simulink library "ddm"  (R2021b)
settings: Solver=VariableStepAuto  StartTime=0.0  StopTime=10.0  RelTol=1e-3
undefined symbols (not defined in the file): ADDM_FrTMTqDev_X_Nm, ADDM_RrTMTqDev_X_Nm, ENUM_ADASACCSTA_ERROR, ENUM_ADASACCSTA_OFF, ENUM_ADASACCSTA_STANDBY, ENUM_ALLOWMOV_ALLOWREADY, ENUM_APS, ENUM_BRKSTA_ERROR, ENUM_BRKSTA_OFF, ENUM_BRKSTA_ON, ENUM_BRKSW_INVALID, ENUM_BRKSW_OFF, ENUM_BRKSW_ON, ENUM_CHGPREACTERRSTA_OBCPRE, ENUM_DCDCFAULTSTA_ANYFAULTLV1, ENUM_DCDCFAULTSTA_ANYFAULTLV2, ENUM_DRIVETRAIN_AWD, ENUM_DRIVETRAIN_FWD, ENUM_DRIVETRAIN_RWD, ENUM_EDUDRTSTA_NORMAL, ENUM_EPBERROR_FAILED, ENUM_EPBSTA_APPLIED, ENUM_EPBSTA_RELEASED, ENUM_ESCAPSSta_APSUNAVAILABLE, ENUM_GEARACTUALPOSN_INVALID, ENUM_GEARACTUALPOSN_P, ENUM_HVBATTREADYPRE_READY, ENUM_HWRESETSTA_HWRESETING, ENUM_MCUWARN_LV0, ENUM_MCUWARN_LV1, ENUM_MCUWARN_LV2, ENUM_MCUWARN_LV3, ENUM_MCUWARN_NOERROR, ENUM_OBCFAULTSTA_ANYFAULT, ENUM_PAS_R2F2, ENUM_PDFAULT_BATTPDFAIL, ENUM_PDFAULT_DCDCDISABLE, ENUM_PDFAULT_MCUDISABLE, ENUM_PDFAULT_MCUDISCHRG, ENUM_POWERSTA_OFF, ENUM_POWERSTA_ON, ENUM_POWERSTA_READY, ENUM_POWERSTA_STANDBY, ENUM_PRESSINDI_LOW, ENUM_PUFAULT_BATTUPFAIL, ENUM_PUFAULT_DCDCENABLEFAIL, ENUM_PUFAULT_PRECHRGCHKFAIL, ENUM_PUFAULT_SAFETYCHKFAIL, ENUM_PWRSTASW_OFF, ENUM_PWRSTASW_OFFA, ENUM_PWRSTASW_OFFCHVCHRG, ENUM_PWRSTASW_OFFCLVCHRG, ENUM_PWRSTASW_ON, ENUM_PWRSTASW_ONHVCHRG, ENUM_PWRSTASW_READY, ENUM_PWRSTASW_STANDBY, ENUM_RAPSErrWarnSta_NORMAL, ENUM_RAPSErrWarnSta_RAPSERRLV1, ENUM_SHIFTCOMMAND_P, ENUM_SHIFTERERRSTA_PBUTTONFAILURE ... (+471)
libraries: hcu_lib x540, simulink x3
(part 22 of 26)

== system ddm/DDM/DDM/PMM/power up and power down/BMS ready fail ==
  note: Test Pass Criteria
  note: Release Condition After Decision
  note: Diagnostics and Fault Handling
  note: Test Detection Criteria
  task_time_s : Inport
  VPMM_PowerSta_enum : Inport  Port=2
  VPMM_PwrStaSW_enum : Inport  Port=3
  VINP_BMSREADY_flg : Inport  Port=4
  VPMM_PowerUpFault_enum : Inport  Port=5
  DTC_clear_request : Inport  Port=6
  Constant : Constant  Value=ENUM_PUFAULT_BATTUPFAIL
  Constant1 : Constant  Value=ENUM_PWRSTASW_OFF
  Constant12 : Constant  Value=ENUM_PWRSTASW_OFF
  Constant13 : Constant  Value=FALSE
  Constant14 : Constant  Value=ZERO_INT
  Constant17 : Constant  Value=KDDM_PwrUpDnDiagnosisOffSW_flg
  Constant18 : Constant  Value=KDDM_BMSRdyPassTO_s
  Constant22 : Constant  Value=ENUM_POWERSTA_OFF
  Constant26 : Constant  Value=KDDM_BMSRdyDTC_cnt
  Constant28 : Constant  Value=KDDM_BMSRdyDTC_cnt
  Constant29 : Constant  Value=FALSE
  Constant41 : Constant  Value=KDDM_BMSRdyDetTO_s
  Constant6 : Constant  Value=TRUE
  Constant7 : Constant  Value=ENUM_POWERSTA_STANDBY
  Constant9 : Constant  Value=KDDM_BMSRdyPassTO_s
  DTC_Couter1 : hcu_lib/Basic_Blocks/DTC_Couter
  DTC_Info : hcu_lib/Basic_Blocks/DTC_Info
  Equal1 : RelationalOperator  Operator===  OutDataTypeStr=boolean  RndMeth=Simplest
  Equal2 : RelationalOperator  Operator=~=  OutDataTypeStr=boolean  RndMeth=Simplest
  Equal4 : RelationalOperator  Operator=~=  OutDataTypeStr=boolean  RndMeth=Simplest
  Equal7 : RelationalOperator  OutDataTypeStr=boolean  RndMeth=Simplest
  Equal8 : RelationalOperator  Operator===  OutDataTypeStr=boolean  RndMeth=Simplest
  Equal9 : RelationalOperator  Operator===  OutDataTypeStr=boolean  RndMeth=Simplest
  Logical Operator13 : Logic  Operator=NOT  AllPortsSameDT=off  OutDataTypeStr=boolean
  Logical Operator14 : Logic  Operator=OR  Inputs=4  AllPortsSameDT=off  OutDataTypeStr=boolean
  Logical Operator16 : Logic  AllPortsSameDT=off  OutDataTypeStr=boolean
  Logical Operator4 : Logic  Operator=NOT  AllPortsSameDT=off  OutDataTypeStr=boolean
  Logical Operator5 : Logic  AllPortsSameDT=off  OutDataTypeStr=boolean
  Relational Operator1 : RelationalOperator  Operator=>  OutDataTypeStr=boolean  RndMeth=Simplest
  Switch1 : Switch  Criteria=u2 ~= 0
  Switch3 : Switch  Criteria=u2 ~= 0
  Switch6 : Switch  Criteria=u2 ~= 0
  Terminator : Terminator
  Test Detection Criteria1 : hcu_lib/Basic_Blocks/Test Detection Criteria
  Timer2 : hcu_lib/Basic_Blocks/Timer
  Unit Delay1 : UnitDelay  SampleTime=-1  HasFrameUpgradeWarning=on
  VDDM_BMSRdyDTC_raw32 : Outport
  VDDM_BMSRdyCFS_flg : Outport  Port=2
  wires:
  [VDDM_BMSRdyCFS_flg] -> VDDM_BMSRdyCFS_flg/1
  Constant12/1 -> Equal4/2
  Constant9/1 -> Timer2/4
  [VPMM_PwrStaSW_enum] -> Equal4/1
  Timer2/1 -> Equal7/1
  Switch1/1 -> Logical Operator13/1, Timer2/2
  Constant6/1 -> Switch1/3
  Constant22/1 -> Equal8/2
  Logical Operator16/1 -> Logical Operator14/1
  Equal8/1 -> Logical Operator16/1
  Constant14/1 -> Relational Operator1/2
  Constant28/1 -> Test Detection Criteria1/3
  Constant18/1 -> Equal7/2
  [task_time_s] -> Timer2/3
  Constant41/1 -> Test Detection Criteria1/4
  [VDDM_BMSRdyCFSRls_flg] -> DTC_Couter1/2
  Constant26/1 -> DTC_Couter1/3
  Logical Operator13/1 -> Timer2/1
  Relational Operator1/1 -> Terminator/1  "VDDM_BMSRdyDFS_flg"
  DTC_Couter1/2 -> Relational Operator1/1  "VDDM_BMSRdyDTC_cnt"
  [VDDM_BMSRdyDet_flg] -> DTC_Couter1/1
  Equal9/1 -> Logical Operator16/2
  Switch6/1 -> Test Detection Criteria1/1
  Constant17/1 -> Logical Operator14/4
  [task_time_s] -> Test Detection Criteria1/2
  Unit Delay1/1 -> Equal8/1
  Constant7/1 -> Equal9/2
  Constant29/1 -> Switch6/1
  Constant13/1 -> Switch3/3
  Logical Operator14/1 -> [VDDM_BMSRdyCFSRls_flg]  "VDDM_BMSRdyCFSRls_flg"
  [VDDM_BMSRdyPass_flg] -> Logical Operator14/3
  Test Detection Criteria1/1 -> [VDDM_BMSRdyDet_flg]  "VDDM_BMSRdyDet_flg"
  Equal4/1 -> Switch3/2
  [VPMM_PowerSta_enum] -> Equal9/1
  Switch3/1 -> Switch6/3
  [VDDM_BMSRdyCFSRls_flg] -> Switch6/2
  [VPMM_PowerSta_enum] -> Unit Delay1/1
  DTC_Couter1/1 -> [VDDM_BMSRdyCFS_flg]  "VDDM_BMSRdyCFS_flg"
  [VDDM_BMSRdyChk_flg] -> Switch3/1
  Equal7/1 -> [VDDM_BMSRdyPass_flg]  "VDDM_BMSRdyPass_flg"
  [DTC_clear_request] -> Logical Operator14/2
  Equal2/1 -> Switch1/2
  Logical Operator5/1 -> [VDDM_BMSRdyChk_flg]
  VPMM_PowerUpFault_enum/1 -> Equal1/1
  VINP_BMSREADY_flg/1 -> Logical Operator4/1
  Logical Operator4/1 -> Logical Operator5/1
  Equal1/1 -> Logical Operator5/2
  Constant/1 -> Equal1/2
  DTC_clear_request/1 -> [DTC_clear_request]
  VPMM_PowerSta_enum/1 -> [VPMM_PowerSta_enum]
  VPMM_PwrStaSW_enum/1 -> [VPMM_PwrStaSW_enum]
  task_time_s/1 -> [task_time_s]
  DTC_Info/1 -> VDDM_BMSRdyDTC_raw32/1  "VDDM_BMSRdyDTC_raw32"
  [VDDM_BMSRdyCFS_flg] -> DTC_Info/3
  [VDDM_BMSRdyDet_flg] -> DTC_Info/1
  [VDDM_BMSRdyPass_flg] -> DTC_Info/2
  [DTC_clear_request] -> DTC_Info/4
  Constant1/1 -> Equal2/2
  [VPMM_PwrStaSW_enum] -> Equal2/1
  [VDDM_BMSRdyChk_flg] -> Switch1/1

== system ddm/DDM/DDM/PMM/power up and power down/DCDC disable fail ==
  note: Release Condition After Decision
  note: Test Detection Criteria
  note: Diagnostics and Fault Handling
  note: Test Pass Criteria
  task_time_s : Inport
  VPMM_PowerSta_enum : Inport  Port=2
  VPMM_PwrStaSW_enum : Inport  Port=3
  VPMM_PowerDownFault_enum : Inport  Port=4
  DTC_clear_request : Inport  Port=5
  Constant : Constant  Value=ENUM_PDFAULT_DCDCDISABLE
  Constant1 : Constant  Value=ENUM_PWRSTASW_OFF
  Constant12 : Constant  Value=ENUM_PWRSTASW_OFF
  Constant13 : Constant  Value=FALSE
  Constant14 : Constant  Value=ZERO_INT
  Constant18 : Constant  Value=KDDM_DCDCDisDTC_cnt
  Constant2 : Constant  Value=KDDM_PwrUpDnDiagnosisOffSW_flg
  Constant23 : Constant  Value=TRUE
  Constant26 : Constant  Value=KDDM_DCDCDisDTC_cnt
  Constant29 : Constant  Value=FALSE
  Constant3 : Constant  Value=ENUM_POWERSTA_OFF
  Constant4 : Constant  Value=KDDM_DCDCDisPassTO_s
  Constant41 : Constant  Value=KDDM_DCDCDisDetTO_s
  Constant8 : Constant  Value=ENUM_POWERSTA_STANDBY
  Constant9 : Constant  Value=KDDM_DCDCDisPassTO_s
  DTC_Couter1 : hcu_lib/Basic_Blocks/DTC_Couter
  DTC_Info : hcu_lib/Basic_Blocks/DTC_Info
  Equal1 : RelationalOperator  Operator===  OutDataTypeStr=boolean  RndMeth=Simplest
  Equal10 : RelationalOperator  Operator===  OutDataTypeStr=boolean  RndMeth=Simplest
  Equal2 : RelationalOperator  Operator=~=  OutDataTypeStr=boolean  RndMeth=Simplest
  Equal5 : RelationalOperator  Operator=~=  OutDataTypeStr=boolean  RndMeth=Simplest
  Equal8 : RelationalOperator  OutDataTypeStr=boolean  RndMeth=Simplest
  Equal9 : RelationalOperator  Operator===  OutDataTypeStr=boolean  RndMeth=Simplest
  Logical Operator13 : Logic  Operator=NOT  AllPortsSameDT=off  OutDataTypeStr=boolean
  Logical Operator14 : Logic  Operator=OR  Inputs=4  AllPortsSameDT=off  OutDataTypeStr=boolean
  Logical Operator16 : Logic  AllPortsSameDT=off  OutDataTypeStr=boolean
  Relational Operator1 : RelationalOperator  Operator=>  OutDataTypeStr=boolean  RndMeth=Simplest
  Switch1 : Switch  Criteria=u2 ~= 0
  Switch3 : Switch  Criteria=u2 ~= 0
  Switch6 : Switch  Criteria=u2 ~= 0
  Terminator : Terminator
  Test Detection Criteria1 : hcu_lib/Basic_Blocks/Test Detection Criteria
  Timer2 : hcu_lib/Basic_Blocks/Timer
  Unit Delay1 : UnitDelay  SampleTime=-1  HasFrameUpgradeWarning=on
  VDDM_DCDCDisDTC_raw32 : Outport
  VDDM_DCDCDisCFS_flg : Outport  Port=2
  wires:
  [VDDM_DCDCDisCFS_flg] -> VDDM_DCDCDisCFS_flg/1
  Constant1/1 -> Equal2/2
  Constant23/1 -> Switch1/3
  [VPMM_PwrStaSW_enum] -> Equal2/1
  Equal2/1 -> Switch1/2
  [VDDM_DCDCDisChk_flg] -> Switch1/1
  Constant18/1 -> DTC_Couter1/3
  Timer2/1 -> Equal8/1
  [VPMM_PwrStaSW_enum] -> Equal5/1
  [VDDM_DCDCDisPass_flg] -> Logical Operator14/3
  [VDDM_DCDCDisCFSRls_flg] -> Switch6/2
  Equal9/1 -> Logical Operator16/1
  Constant26/1 -> Test Detection Criteria1/3
  Equal8/1 -> [VDDM_DCDCDisPass_flg]  "VDDM_DCDCDisPass_flg"
  Switch1/1 -> Logical Operator13/1, Timer2/2
  Switch6/1 -> Test Detection Criteria1/1
  Constant41/1 -> Test Detection Criteria1/4
  DTC_Couter1/2 -> Relational Operator1/1  "VDDM_DCDCDisDTC_cnt"
  Equal10/1 -> Logical Operator16/2
  [VDDM_DCDCDisCFSRls_flg] -> DTC_Couter1/2
  Unit Delay1/1 -> Equal9/1
  Constant12/1 -> Equal5/2
  Test Detection Criteria1/1 -> [VDDM_DCDCDisDet_flg]  "VDDM_DCDCDisDet_flg"
  [task_time_s] -> Test Detection Criteria1/2
  [VDDM_DCDCDisDet_flg] -> DTC_Couter1/1
  [task_time_s] -> Timer2/3
  [VPMM_PowerSta_enum] -> Unit Delay1/1
  Constant2/1 -> Logical Operator14/4
  [VPMM_PowerSta_enum] -> Equal10/1
  Constant8/1 -> Equal10/2
  Constant3/1 -> Equal9/2
  Logical Operator13/1 -> Timer2/1
  Logical Operator16/1 -> Logical Operator14/1
  Logical Operator14/1 -> [VDDM_DCDCDisCFSRls_flg]  "VDDM_DCDCDisCFSRls_flg"
  [VDDM_DCDCDisChk_flg] -> Switch3/1
  Relational Operator1/1 -> Terminator/1  "VDDM_DCDCDisDFS_flg"
  Switch3/1 -> Switch6/3
  Constant13/1 -> Switch3/3
  Equal5/1 -> Switch3/2
  Constant29/1 -> Switch6/1
  DTC_Couter1/1 -> [VDDM_DCDCDisCFS_flg]  "VDDM_DCDCDisCFS_flg"
  [DTC_clear_request] -> Logical Operator14/2
  Constant14/1 -> Relational Operator1/2
  Constant4/1 -> Timer2/4
  Constant9/1 -> Equal8/2
  VPMM_PowerSta_enum/1 -> [VPMM_PowerSta_enum]
  VPMM_PwrStaSW_enum/1 -> [VPMM_PwrStaSW_enum]
  task_time_s/1 -> [task_time_s]
  VPMM_PowerDownFault_enum/1 -> Equal1/1
  Constant/1 -> Equal1/2
  DTC_clear_request/1 -> [DTC_clear_request]
  Equal1/1 -> [VDDM_DCDCDisChk_flg]
  DTC_Info/1 -> VDDM_DCDCDisDTC_raw32/1  "VDDM_DCDCDisDTC_raw32"
  [VDDM_DCDCDisPass_flg] -> DTC_Info/2
  [VDDM_DCDCDisCFS_flg] -> DTC_Info/3
  [VDDM_DCDCDisDet_flg] -> DTC_Info/1
  [DTC_clear_request] -> DTC_Info/4

== system ddm/DDM/DDM/PMM/power up and power down/DCDC enable fail ==
  note: Release Condition After Decision
  note: Test Detection Criteria
  note: Test Pass Criteria
  note: Diagnostics and Fault Handling
  task_time_s : Inport
  VPMM_PowerSta_enum : Inport  Port=2
  VPMM_PwrStaSW_enum : Inport  Port=3
  VINP_DCDCEnabled_flg : Inport  Port=4
  VPMM_PowerUpFault_enum : Inport  Port=5
  DTC_clear_request : Inport  Port=6
  Constant : Constant  Value=ENUM_PUFAULT_DCDCENABLEFAIL
  Constant1 : Constant  Value=ENUM_PWRSTASW_OFF
  Constant12 : Constant  Value=ENUM_PWRSTASW_OFF
  Constant13 : Constant  Value=FALSE
  Constant14 : Constant  Value=ZERO_INT
  Constant17 : Constant  Value=KDDM_PwrUpDnDiagnosisOffSW_flg
  Constant18 : Constant  Value=KDDM_DCDCEnaDTC_cnt
  Constant22 : Constant  Value=ENUM_POWERSTA_OFF
  Constant28 : Constant  Value=KDDM_DCDCEnaDTC_cnt
  Constant29 : Constant  Value=FALSE
  Constant3 : Constant  Value=KDDM_DCDCEnaPassTO_s
  Constant41 : Constant  Value=KDDM_DCDCEnaDetTO_s
  Constant6 : Constant  Value=TRUE
  Constant7 : Constant  Value=ENUM_POWERSTA_STANDBY
  Constant9 : Constant  Value=KDDM_DCDCEnaPassTO_s
  DTC_Couter1 : hcu_lib/Basic_Blocks/DTC_Couter
  DTC_Info : hcu_lib/Basic_Blocks/DTC_Info
  Equal1 : RelationalOperator  Operator===  OutDataTypeStr=boolean  RndMeth=Simplest
  Equal2 : RelationalOperator  Operator=~=  OutDataTypeStr=boolean  RndMeth=Simplest
  Equal4 : RelationalOperator  Operator=~=  OutDataTypeStr=boolean  RndMeth=Simplest
  Equal7 : RelationalOperator  OutDataTypeStr=boolean  RndMeth=Simplest
  Equal8 : RelationalOperator  Operator===  OutDataTypeStr=boolean  RndMeth=Simplest
  Equal9 : RelationalOperator  Operator===  OutDataTypeStr=boolean  RndMeth=Simplest
  Logical Operator13 : Logic  Operator=NOT  AllPortsSameDT=off  OutDataTypeStr=boolean
  Logical Operator14 : Logic  Operator=OR  Inputs=4  AllPortsSameDT=off  OutDataTypeStr=boolean
  Logical Operator16 : Logic  AllPortsSameDT=off  OutDataTypeStr=boolean
  Logical Operator4 : Logic  Operator=NOT  AllPortsSameDT=off  OutDataTypeStr=boolean
  Logical Operator5 : Logic  AllPortsSameDT=off  OutDataTypeStr=boolean
  Relational Operator1 : RelationalOperator  Operator=>  OutDataTypeStr=boolean  RndMeth=Simplest
  Switch1 : Switch  Criteria=u2 ~= 0
  Switch3 : Switch  Criteria=u2 ~= 0
  Switch6 : Switch  Criteria=u2 ~= 0
  Terminator : Terminator
  Test Detection Criteria1 : hcu_lib/Basic_Blocks/Test Detection Criteria
  Timer2 : hcu_lib/Basic_Blocks/Timer
  Unit Delay1 : UnitDelay  SampleTime=-1  HasFrameUpgradeWarning=on
  VDDM_DCDCEnaDTC_raw32 : Outport
  VDDM_DCDCEnaCFS_flg : Outport  Port=2
  wires:
  [VDDM_DCDCEnaCFS_flg] -> VDDM_DCDCEnaCFS_flg/1
  Constant6/1 -> Switch1/3
  Logical Operator13/1 -> Timer2/1
  Logical Operator16/1 -> Logical Operator14/1
  Timer2/1 -> Equal7/1
  [VPMM_PwrStaSW_enum] -> Equal4/1
  Logical Operator14/1 -> [VDDM_DCDCEnaCFSRls_flg]  "VDDM_DCDCEnaCFSRls_flg"
  Equal8/1 -> Logical Operator16/1
  Constant18/1 -> DTC_Couter1/3
  Constant41/1 -> Test Detection Criteria1/4
  DTC_Couter1/2 -> Relational Operator1/1  "VDDM_DCDCEnaDTC_cnt"
  Relational Operator1/1 -> Terminator/1  "VDDM_DCDCEnaDFS_flg"
  [task_time_s] -> Timer2/3
  [VDDM_DCDCEnaChk_flg] -> Switch3/1
  [VPMM_PowerSta_enum] -> Unit Delay1/1
  Constant22/1 -> Equal8/2
  Constant28/1 -> Test Detection Criteria1/3
  Constant13/1 -> Switch3/3
  Switch6/1 -> Test Detection Criteria1/1
  DTC_Couter1/1 -> [VDDM_DCDCEnaCFS_flg]  "VDDM_DCDCEnaCFS_flg"
  Equal9/1 -> Logical Operator16/2
  [task_time_s] -> Test Detection Criteria1/2
  Constant3/1 -> Timer2/4
  Constant17/1 -> Logical Operator14/4
  Equal4/1 -> Switch3/2
  [VDDM_DCDCEnaCFSRls_flg] -> Switch6/2
  Unit Delay1/1 -> Equal8/1
  [VPMM_PowerSta_enum] -> Equal9/1
  Constant7/1 -> Equal9/2
  Constant29/1 -> Switch6/1
  [VDDM_DCDCEnaPass_flg] -> Logical Operator14/3
  Constant12/1 -> Equal4/2
  [DTC_clear_request] -> Logical Operator14/2
  Switch1/1 -> Logical Operator13/1, Timer2/2
  Switch3/1 -> Switch6/3
  Constant14/1 -> Relational Operator1/2
  Constant9/1 -> Equal7/2
  Equal7/1 -> [VDDM_DCDCEnaPass_flg]  "VDDM_DCDCEnaPass_flg"
  [VDDM_DCDCEnaDet_flg] -> DTC_Couter1/1
  Test Detection Criteria1/1 -> [VDDM_DCDCEnaDet_flg]  "VDDM_DCDCEnaDet_flg"
  [VDDM_DCDCEnaCFSRls_flg] -> DTC_Couter1/2
  task_time_s/1 -> [task_time_s]
  VPMM_PwrStaSW_enum/1 -> [VPMM_PwrStaSW_enum]
  VPMM_PowerSta_enum/1 -> [VPMM_PowerSta_enum]
  DTC_clear_request/1 -> [DTC_clear_request]
  Constant/1 -> Equal1/2
  Equal1/1 -> Logical Operator5/2
  Logical Operator4/1 -> Logical Operator5/1
  VINP_DCDCEnabled_flg/1 -> Logical Operator4/1
  VPMM_PowerUpFault_enum/1 -> Equal1/1
  Logical Operator5/1 -> [VDDM_DCDCEnaChk_flg]
  DTC_Info/1 -> VDDM_DCDCEnaDTC_raw32/1  "VDDM_DCDCEnaDTC_raw32"
  [VDDM_DCDCEnaPass_flg] -> DTC_Info/2
  [VDDM_DCDCEnaCFS_flg] -> DTC_Info/3
  [VDDM_DCDCEnaDet_flg] -> DTC_Info/1
  [DTC_clear_request] -> DTC_Info/4
  [VPMM_PwrStaSW_enum] -> Equal2/1
  Constant1/1 -> Equal2/2
  [VDDM_DCDCEnaChk_flg] -> Switch1/1
  Equal2/1 -> Switch1/2

== system ddm/DDM/DDM/PMM/power up and power down/DCDC ready for precharge fail ==
  note: Diagnostics and Fault Handling
  note: Test Detection Criteria
  note: Release Condition After Decision
  note: Test Pass Criteria
  task_time_s : Inport
  VPMM_PowerSta_enum : Inport  Port=2
  VPMM_PwrStaSW_enum : Inport  Port=3
  VINP_DCDCReady4Pre_flg : Inport  Port=4
  VPMM_PowerUpFault_enum : Inport  Port=5
  VINP_ReqClrDTC_flg : Inport  Port=6
  Constant : Constant  Value=ENUM_PUFAULT_PRECHRGCHKFAIL
  Constant1 : Constant  Value=ENUM_PWRSTASW_OFF
  Constant12 : Constant  Value=ENUM_PWRSTASW_OFF
  Constant13 : Constant  Value=FALSE
  Constant14 : Constant  Value=ZERO_INT
  Constant17 : Constant  Value=KDDM_PwrUpDnDiagnosisOffSW_flg
  Constant18 : Constant  Value=KDDM_DCDC4PrePassTO_s
  Constant22 : Constant  Value=ENUM_POWERSTA_OFF
  Constant28 : Constant  Value=KDDM_DCDC4PrePassTO_s
  Constant29 : Constant  Value=FALSE
  Constant3 : Constant  Value=KDDM_DCDC4PreDTC_cnt
  Constant41 : Constant  Value=KDDM_DCDC4PreDetTO_s
  Constant6 : Constant  Value=TRUE
  Constant7 : Constant  Value=ENUM_POWERSTA_STANDBY
  Constant9 : Constant  Value=KDDM_DCDC4PreDTC_cnt
  DTC_Couter1 : hcu_lib/Basic_Blocks/DTC_Couter
  DTC_Info : hcu_lib/Basic_Blocks/DTC_Info
  Equal1 : RelationalOperator  Operator===  OutDataTypeStr=boolean  RndMeth=Simplest
  Equal2 : RelationalOperator  Operator=~=  OutDataTypeStr=boolean  RndMeth=Simplest
  Equal4 : RelationalOperator  Operator=~=  OutDataTypeStr=boolean  RndMeth=Simplest
  Equal7 : RelationalOperator  OutDataTypeStr=boolean  RndMeth=Simplest
  Equal8 : RelationalOperator  Operator===  OutDataTypeStr=boolean  RndMeth=Simplest
  Equal9 : RelationalOperator  Operator===  OutDataTypeStr=boolean  RndMeth=Simplest
  Logical Operator13 : Logic  Operator=NOT  AllPortsSameDT=off  OutDataTypeStr=boolean
  Logical Operator14 : Logic  Operator=OR  Inputs=4  AllPortsSameDT=off  OutDataTypeStr=boolean
  Logical Operator16 : Logic  AllPortsSameDT=off  OutDataTypeStr=boolean
  Logical Operator4 : Logic  Operator=NOT  AllPortsSameDT=off  OutDataTypeStr=boolean
  Logical Operator5 : Logic  AllPortsSameDT=off  OutDataTypeStr=boolean
  Relational Operator1 : RelationalOperator  Operator=>  OutDataTypeStr=boolean  RndMeth=Simplest
  Switch1 : Switch  Criteria=u2 ~= 0
  Switch3 : Switch  Criteria=u2 ~= 0
  Switch6 : Switch  Criteria=u2 ~= 0
  Terminator : Terminator
  Test Detection Criteria1 : hcu_lib/Basic_Blocks/Test Detection Criteria
  Timer2 : hcu_lib/Basic_Blocks/Timer
  Unit Delay1 : UnitDelay  SampleTime=-1  HasFrameUpgradeWarning=on
  VDDM_DCDC4PreDTC_raw32 : Outport
  VDDM_DCDC4PreCFS_flg : Outport  Port=2
  wires:
  [VDDM_DCDC4PreCFS_flg] -> VDDM_DCDC4PreCFS_flg/1
  Logical Operator13/1 -> Timer2/1
  [VDDM_DCDC4PreChk_flg] -> Switch3/1
  Constant17/1 -> Logical Operator14/4
  Constant28/1 -> Equal7/2
  [VDDM_DCDC4PreCFSRls_flg] -> Switch6/2
  Constant3/1 -> DTC_Couter1/3
  Equal7/1 -> [VDDM_DCDC4PrePass_flg]  "VDDM_DCDC4PrePass_flg"
  Relational Operator1/1 -> Terminator/1  "VDDM_DCDC4PreDFS_flg"
  Logical Operator14/1 -> [VDDM_DCDC4PreCFSRls_flg]  "VDDM_DCDC4PreCFSRls_flg"
  Equal8/1 -> Logical Operator16/1
  DTC_Couter1/1 -> [VDDM_DCDC4PreCFS_flg]  "VDDM_DCDC4PreCFS_flg"
  [VDDM_DCDC4PreDet_flg] -> DTC_Couter1/1
  Constant41/1 -> Test Detection Criteria1/4
  [VPMM_PwrStaSW_enum] -> Equal4/1
  Constant13/1 -> Switch3/3
  Timer2/1 -> Equal7/1
  Logical Operator16/1 -> Logical Operator14/1
  Constant6/1 -> Switch1/3
  [VDDM_DCDC4PrePass_flg] -> Logical Operator14/3
  Constant12/1 -> Equal4/2
  Equal2/1 -> Switch1/2
  Switch1/1 -> Logical Operator13/1, Timer2/2
  Constant14/1 -> Relational Operator1/2
  Switch3/1 -> Switch6/3
  [DTC_clear_request] -> Logical Operator14/2
  Constant29/1 -> Switch6/1
  Equal4/1 -> Switch3/2
  [VPMM_PowerSta_enum] -> Equal9/1
  Constant7/1 -> Equal9/2
  [VDDM_DCDC4PreCFSRls_flg] -> DTC_Couter1/2
  Unit Delay1/1 -> Equal8/1
  [task_time_s] -> Test Detection Criteria1/2
  Equal9/1 -> Logical Operator16/2
  Switch6/1 -> Test Detection Criteria1/1
  Constant9/1 -> Test Detection Criteria1/3
  [task_time_s] -> Timer2/3
  [VPMM_PowerSta_enum] -> Unit Delay1/1
  Constant22/1 -> Equal8/2
  DTC_Couter1/2 -> Relational Operator1/1  "VDDM_DCDC4PreDTC_cnt"
  Test Detection Criteria1/1 -> [VDDM_DCDC4PreDet_flg]  "VDDM_DCDC4PreDet_flg"
  Constant18/1 -> Timer2/4
  VPMM_PowerSta_enum/1 -> [VPMM_PowerSta_enum]
  VPMM_PwrStaSW_enum/1 -> [VPMM_PwrStaSW_enum]
  task_time_s/1 -> [task_time_s]
  VINP_ReqClrDTC_flg/1 -> [DTC_clear_request]
  Equal1/1 -> Logical Operator5/2
  Constant/1 -> Equal1/2
  VPMM_PowerUpFault_enum/1 -> Equal1/1
  Logical Operator5/1 -> [VDDM_DCDC4PreChk_flg]
  VINP_DCDCReady4Pre_flg/1 -> Logical Operator4/1
  Logical Operator4/1 -> Logical Operator5/1
  DTC_Info/1 -> VDDM_DCDC4PreDTC_raw32/1  "VDDM_DCDC4PreDTC_raw32"
  [VDDM_DCDC4PrePass_flg] -> DTC_Info/2
  [VDDM_DCDC4PreCFS_flg] -> DTC_Info/3
  [VDDM_DCDC4PreDet_flg] -> DTC_Info/1
  [DTC_clear_request] -> DTC_Info/4
  Constant1/1 -> Equal2/2
  [VDDM_DCDC4PreChk_flg] -> Switch1/1
  [VPMM_PwrStaSW_enum] -> Equal2/1

== system ddm/DDM/DDM/PMM/power up and power down/Fr_MCU active discharge fail ==
  note: Diagnostics and Fault Handling
  note: Release Condition After Decision
  note: Test Detection Criteria
  note: Test Pass Criteria
  task_time_s : Inport
  VPMM_PowerSta_enum : Inport  Port=2
  VPMM_PwrStaSW_enum : Inport  Port=3
  VPMM_PowerDownFault_enum : Inport  Port=4
  DTC_clear_request : Inport  Port=5
  VDDM_FrMCUDCBusVolt_V : Inport  Port=6
  Constant : Constant  Value=ENUM_PDFAULT_MCUDISCHRG
  Constant1 : Constant  Value=FALSE
  Constant10 : Constant  Value=KDDM_MCUDischrgVolt_V
  Constant12 : Constant  Value=ENUM_PWRSTASW_OFF
  Constant13 : Constant  Value=FALSE
  Constant14 : Constant  Value=ZERO_INT
  Constant18 : Constant  Value=KDDM_MCUDischrgVolt_V
  Constant19 : Constant  Value=KDDM_FrMCUActDTC_cnt
  Constant2 : Constant  Value=TRUE
  Constant26 : Constant  Value=KDDM_FrMCUActDTC_cnt
  Constant29 : Constant  Value=FALSE
  Constant3 : Constant  Value=KDDM_PwrUpDnDiagnosisOffSW_flg
  Constant4 : Constant  Value=ENUM_POWERSTA_OFF
  Constant41 : Constant  Value=KDDM_FrMCUActDetTO_s
  Constant5 : Constant  Value=ENUM_PWRSTASW_OFF
  Constant6 : Constant  Value=TRUE
  Constant7 : Constant  Value=KDDM_FrMCUActPassTO_s
  Constant8 : Constant  Value=KDDM_FrMCUActPassTO_s
  Constant9 : Constant  Value=ENUM_POWERSTA_STANDBY
  DTC_Couter1 : hcu_lib/Basic_Blocks/DTC_Couter
  DTC_Info : hcu_lib/Basic_Blocks/DTC_Info
  Equal1 : RelationalOperator  Operator===  OutDataTypeStr=boolean  RndMeth=Simplest
  Equal11 : RelationalOperator  Operator=<=  OutDataTypeStr=boolean  RndMeth=Simplest
  Equal2 : RelationalOperator  Operator=>  OutDataTypeStr=boolean  RndMeth=Simplest
  Equal3 : RelationalOperator  Operator===  OutDataTypeStr=boolean  RndMeth=Simplest
  Equal5 : RelationalOperator  Operator=~=  OutDataTypeStr=boolean  RndMeth=Simplest
  Equal7 : RelationalOperator  Operator=~=  OutDataTypeStr=boolean  RndMeth=Simplest
  Equal8 : RelationalOperator  OutDataTypeStr=boolean  RndMeth=Simplest
  Equal9 : RelationalOperator  Operator===  OutDataTypeStr=boolean  RndMeth=Simplest
  Logical Operator13 : Logic  Operator=NOT  AllPortsSameDT=off  OutDataTypeStr=boolean
  Logical Operator14 : Logic  Operator=OR  Inputs=5  AllPortsSameDT=off  OutDataTypeStr=boolean
  Logical Operator16 : Logic  AllPortsSameDT=off  OutDataTypeStr=boolean
  Logical Operator4 : Logic  AllPortsSameDT=off  OutDataTypeStr=boolean
  Relational Operator1 : RelationalOperator  Operator=>  OutDataTypeStr=boolean  RndMeth=Simplest
  Switch{1..3,6} (4 alike) : Switch  Criteria=u2 ~= 0
  Terminator : Terminator
  Test Detection Criteria1 : hcu_lib/Basic_Blocks/Test Detection Criteria
  Timer2 : hcu_lib/Basic_Blocks/Timer
  Unit Delay1 : UnitDelay  SampleTime=-1  HasFrameUpgradeWarning=on
  VDDM_FrMCUActDTC_raw32 : Outport
  VDDM_FrMCUActDisFail_flg : Outport  Port=2
  VDDM_FrMCUActCFS_flg : Outport  Port=3
  wires:
  [VDDM_FrMCUDCBusVolt_V] -> Equal2/1
  Constant10/1 -> Equal2/2
  Equal2/1 -> Logical Operator4/1
  Equal1/1 -> Logical Operator4/2
  Logical Operator4/1 -> [VDDM_FrMCUActChk_flg]
  VDDM_FrMCUDCBusVolt_V/1 -> [VDDM_FrMCUDCBusVolt_V]
  [DTC_clear_request] -> DTC_Info/4
  [VDDM_FrMCUActDet_flg] -> DTC_Info/1
  [VDDM_FrMCUActCFS_flg] -> DTC_Info/3
  [VDDM_FrMCUActPass_flg] -> DTC_Info/2
  DTC_Info/1 -> VDDM_FrMCUActDTC_raw32/1  "VDDM_FrMCUActDTC_raw32"
  VPMM_PowerDownFault_enum/1 -> Equal1/1
  Constant/1 -> Equal1/2
  DTC_clear_request/1 -> [DTC_clear_request]
  task_time_s/1 -> [task_time_s]
  VPMM_PwrStaSW_enum/1 -> [VPMM_PwrStaSW_enum]
  VPMM_PowerSta_enum/1 -> [VPMM_PowerSta_enum]
  DTC_Couter1/1 -> [VDDM_FrMCUActCFS_flg]  "VDDM_FrMCUActCFS_flg"
  Equal5/1 -> Switch2/2
  [VPMM_PwrStaSW_enum] -> Equal5/1
  [VDDM_FrMCUActChk_flg] -> Switch2/1
  Equal8/1 -> [VDDM_FrMCUActPass_flg]  "VDDM_FrMCUActPass_flg"
  [VDDM_FrMCUActCFSRls_flg] -> Switch6/2
  Constant6/1 -> Switch2/3
  Equal7/1 -> Switch3/2
  [VDDM_FrMCUActDet_flg] -> DTC_Couter1/1
  Constant26/1 -> Test Detection Criteria1/3
  Logical Operator14/1 -> [VDDM_FrMCUActCFSRls_flg]  "VDDM_FrMCUActCFSRls_flg"
  Constant8/1 -> Equal8/2
  Constant13/1 -> Switch3/3
  Constant14/1 -> Relational Operator1/2
  Equal3/1 -> Logical Operator16/2
  Constant5/1 -> Equal5/2
  Switch6/1 -> Test Detection Criteria1/1
  [task_time_s] -> Test Detection Criteria1/2
  Constant29/1 -> Switch6/1
  Switch2/1 -> Timer2/2, Logical Operator13/1
  Constant19/1 -> DTC_Couter1/3
  Constant3/1 -> Logical Operator14/5
  Equal9/1 -> Logical Operator16/1
  [task_time_s] -> Timer2/3
  [VDDM_FrMCUActChk_flg] -> Switch3/1
  Logical Operator13/1 -> Timer2/1
  Switch3/1 -> Switch6/3
  Constant9/1 -> Equal3/2
  Unit Delay1/1 -> Equal9/1
  [VPMM_PowerSta_enum] -> Equal3/1
  [VDDM_FrMCUActCFSRls_flg] -> DTC_Couter1/2
  [DTC_clear_request] -> Logical Operator14/2
  Constant4/1 -> Equal9/2
  DTC_Couter1/2 -> Relational Operator1/1  "VDDM_FrMCUActDTC_cnt"
  Timer2/1 -> Equal8/1
  [VPMM_PwrStaSW_enum] -> Equal7/1
  [VPMM_PowerSta_enum] -> Unit Delay1/1
  Logical Operator16/1 -> Logical Operator14/1
  Constant41/1 -> Test Detection Criteria1/4
  Constant7/1 -> Timer2/4
  Relational Operator1/1 -> Terminator/1  "VDDM_FrMCUActDFS_flg"
  Constant12/1 -> Equal7/2
  Test Detection Criteria1/1 -> [VDDM_FrMCUActDet_flg]  "VDDM_FrMCUActDet_flg"
  [VDDM_FrMCUDCBusVolt_V] -> Equal11/1
  Equal11/1 -> Logical Operator14/4
  Constant18/1 -> Equal11/2
  [VDDM_FrMCUActPass_flg] -> Logical Operator14/3
  Constant2/1 -> Switch1/1
  Constant1/1 -> Switch1/3
  [VDDM_FrMCUActCFS_flg] -> VDDM_FrMCUActCFS_flg/1, Switch1/2
  Switch1/1 -> VDDM_FrMCUActDisFail_flg/1  "VDDM_FrMCUActDisFail_flg"

== system ddm/DDM/DDM/PMM/power up and power down/Fr_MCU disable fail ==
  note: Test Detection Criteria
  note: Test Pass Criteria
  note: Diagnostics and Fault Handling
  note: Release Condition After Decision
  task_time_s : Inport
  VPMM_PowerSta_enum : Inport  Port=2
  VPMM_PwrStaSW_enum : Inport  Port=3
  VPMM_PowerDownFault_enum : Inport  Port=4
  DTC_clear_request : Inport  Port=5
  VDDM_FrMCUEnaSta_flg : Inport  Port=6
  Constant : Constant  Value=ENUM_PDFAULT_MCUDISABLE
  Constant1 : Constant  Value=KDDM_PwrUpDnDiagnosisOffSW_flg
  Constant12 : Constant  Value=ENUM_PWRSTASW_OFF
  Constant13 : Constant  Value=FALSE
  Constant14 : Constant  Value=ZERO_INT
  Constant18 : Constant  Value=KDDM_FrMCUDisDTC_cnt
  Constant2 : Constant  Value=ENUM_PWRSTASW_OFF
  Constant23 : Constant  Value=TRUE
  Constant26 : Constant  Value=KDDM_FrMCUDisDTC_cnt
  Constant29 : Constant  Value=FALSE
  Constant3 : Constant  Value=ENUM_POWERSTA_OFF
  Constant4 : Constant  Value=KDDM_FrMCUDisPassTO_s
  Constant41 : Constant  Value=KDDM_FrMCUDisDetTO_s
  Constant8 : Constant  Value=ENUM_POWERSTA_STANDBY
  Constant9 : Constant  Value=KDDM_FrMCUDisPassTO_s
  DTC_Couter1 : hcu_lib/Basic_Blocks/DTC_Couter
  DTC_Info : hcu_lib/Basic_Blocks/DTC_Info
  Equal1 : RelationalOperator  Operator===  OutDataTypeStr=boolean  RndMeth=Simplest
  Equal10 : RelationalOperator  Operator===  OutDataTypeStr=boolean  RndMeth=Simplest
  Equal2 : RelationalOperator  Operator=~=  OutDataTypeStr=boolean  RndMeth=Simplest
  Equal5 : RelationalOperator  Operator=~=  OutDataTypeStr=boolean  RndMeth=Simplest
  Equal8 : RelationalOperator  OutDataTypeStr=boolean  RndMeth=Simplest
  Equal9 : RelationalOperator  Operator===  OutDataTypeStr=boolean  RndMeth=Simplest
  Logical Operator13 : Logic  Operator=NOT  AllPortsSameDT=off  OutDataTypeStr=boolean
  Logical Operator14 : Logic  Operator=OR  Inputs=4  AllPortsSameDT=off  OutDataTypeStr=boolean
  Logical Operator16 : Logic  AllPortsSameDT=off  OutDataTypeStr=boolean
  Logical Operator4 : Logic  AllPortsSameDT=off  OutDataTypeStr=boolean
  Relational Operator1 : RelationalOperator  Operator=>  OutDataTypeStr=boolean  RndMeth=Simplest
  Switch1 : Switch  Criteria=u2 ~= 0
  Switch3 : Switch  Criteria=u2 ~= 0
  Switch6 : Switch  Criteria=u2 ~= 0
  Terminator : Terminator
  Test Detection Criteria1 : hcu_lib/Basic_Blocks/Test Detection Criteria
  Timer2 : hcu_lib/Basic_Blocks/Timer
  Unit Delay1 : UnitDelay  SampleTime=-1  HasFrameUpgradeWarning=on
  VDDM_FrMCUDisDTC_raw32 : Outport
  VDDM_FrMCUDisCFS_flg : Outport  Port=2
  wires:
  [VDDM_FrMCUDisCFS_flg] -> VDDM_FrMCUDisCFS_flg/1
  Constant23/1 -> Switch1/3
  [VDDM_FrMCUDisChk_flg] -> Switch1/1
  Equal2/1 -> Switch1/2
  Constant2/1 -> Equal2/2
  [VPMM_PwrStaSW_enum] -> Equal2/1
  DTC_Couter1/1 -> [VDDM_FrMCUDisCFS_flg]  "VDDM_FrMCUDisCFS_flg"
  [VPMM_PwrStaSW_enum] -> Equal5/1
  Equal8/1 -> [VDDM_FrMCUDisPass_flg]  "VDDM_FrMCUDisPass_flg"
  [task_time_s] -> Test Detection Criteria1/2
  Constant26/1 -> Test Detection Criteria1/3
  Unit Delay1/1 -> Equal9/1
  [VDDM_FrMCUDisChk_flg] -> Switch3/1
  Test Detection Criteria1/1 -> [VDDM_FrMCUDisDet_flg]  "VDDM_FrMCUDisDet_flg"
  Equal10/1 -> Logical Operator16/2
  DTC_Couter1/2 -> Relational Operator1/1  "VDDM_FrMCUDisDTC_cnt"
  Switch6/1 -> Test Detection Criteria1/1
  Constant4/1 -> Timer2/4
  Switch1/1 -> Logical Operator13/1, Timer2/2
  Logical Operator14/1 -> [VDDM_FrMCUDisCFSRls_flg]  "VDDM_FrMCUDisCFSRls_flg"
  Switch3/1 -> Switch6/3
  Constant13/1 -> Switch3/3
  Constant14/1 -> Relational Operator1/2
  [VDDM_FrMCUDisPass_flg] -> Logical Operator14/3
  [DTC_clear_request] -> Logical Operator14/2
  Constant29/1 -> Switch6/1
  Equal5/1 -> Switch3/2
  Constant9/1 -> Equal8/2
  [VDDM_FrMCUDisCFSRls_flg] -> DTC_Couter1/2
  Constant41/1 -> Test Detection Criteria1/4
  Logical Operator16/1 -> Logical Operator14/1
  Constant12/1 -> Equal5/2
  Logical Operator13/1 -> Timer2/1
  Equal9/1 -> Logical Operator16/1
  Timer2/1 -> Equal8/1
  Constant18/1 -> DTC_Couter1/3
  Constant1/1 -> Logical Operator14/4
  [VPMM_PowerSta_enum] -> Unit Delay1/1
  [VPMM_PowerSta_enum] -> Equal10/1
  Constant3/1 -> Equal9/2
  Constant8/1 -> Equal10/2
  [task_time_s] -> Timer2/3
  [VDDM_FrMCUDisDet_flg] -> DTC_Couter1/1
  Relational Operator1/1 -> Terminator/1  "VDDM_FrMCUDisDFS_flg"
  [VDDM_FrMCUDisCFSRls_flg] -> Switch6/2
  task_time_s/1 -> [task_time_s]
  VPMM_PwrStaSW_enum/1 -> [VPMM_PwrStaSW_enum]
  VPMM_PowerSta_enum/1 -> [VPMM_PowerSta_enum]
  Constant/1 -> Equal1/2
  VPMM_PowerDownFault_enum/1 -> Equal1/1
  DTC_clear_request/1 -> [DTC_clear_request]
  DTC_Info/1 -> VDDM_FrMCUDisDTC_raw32/1  "VDDM_FrMCUDisDTC_raw32"
  [VDDM_FrMCUDisPass_flg] -> DTC_Info/2
  [VDDM_FrMCUDisCFS_flg] -> DTC_Info/3
  [VDDM_FrMCUDisDet_flg] -> DTC_Info/1
  [DTC_clear_request] -> DTC_Info/4
  VDDM_FrMCUEnaSta_flg/1 -> [VDDM_FrMCUEnaSta_flg]
  Logical Operator4/1 -> [VDDM_FrMCUDisChk_flg]  "VDDM_FrMCUDisChk_flg"
  Equal1/1 -> Logical Operator4/2
  [VDDM_FrMCUEnaSta_flg] -> Logical Operator4/1

== system ddm/DDM/DDM/PMM/power up and power down/Fr_MCU ready for precharge fail ==
  note: Diagnostics and Fault Handling
  note: Test Detection Criteria
  note: Test Pass Criteria
  note: Release Condition After Decision
  task_time_s : Inport
  VPMM_PowerSta_enum : Inport  Port=2
  VPMM_PwrStaSW_enum : Inport  Port=3
  VPMM_PowerUpFault_enum : Inport  Port=4
  DTC_clear_request : Inport  Port=5
  VDDM_FrMCUReady4Pre_flg : Inport  Port=6
  Constant : Constant  Value=ENUM_PUFAULT_PRECHRGCHKFAIL
  Constant1 : Constant  Value=ENUM_PWRSTASW_OFF
  Constant12 : Constant  Value=ENUM_PWRSTASW_OFF
  Constant13 : Constant  Value=FALSE
  Constant14 : Constant  Value=ZERO_INT
  Constant17 : Constant  Value=KDDM_PwrUpDnDiagnosisOffSW_flg
  Constant18 : Constant  Value=KDDM_FrMCU4PrePassTO_s
  Constant22 : Constant  Value=ENUM_POWERSTA_OFF
  Constant28 : Constant  Value=KDDM_FrMCU4PrePassTO_s
  Constant29 : Constant  Value=FALSE
  Constant3 : Constant  Value=KDDM_FrMCU4PreDTC_cnt
  Constant41 : Constant  Value=KDDM_FrMCU4PreDetTO_s
  Constant6 : Constant  Value=TRUE
  Constant7 : Constant  Value=ENUM_POWERSTA_STANDBY
  Constant9 : Constant  Value=KDDM_FrMCU4PreDTC_cnt
  DTC_Couter1 : hcu_lib/Basic_Blocks/DTC_Couter
  DTC_Info : hcu_lib/Basic_Blocks/DTC_Info
  Equal1 : RelationalOperator  Operator===  OutDataTypeStr=boolean  RndMeth=Simplest
  Equal2 : RelationalOperator  Operator=~=  OutDataTypeStr=boolean  RndMeth=Simplest
  Equal4 : RelationalOperator  Operator=~=  OutDataTypeStr=boolean  RndMeth=Simplest
  Equal7 : RelationalOperator  OutDataTypeStr=boolean  RndMeth=Simplest
  Equal8 : RelationalOperator  Operator===  OutDataTypeStr=boolean  RndMeth=Simplest
  Equal9 : RelationalOperator  Operator===  OutDataTypeStr=boolean  RndMeth=Simplest
  Logical Operator1 : Logic  Operator=NOT  AllPortsSameDT=off  OutDataTypeStr=boolean
  Logical Operator13 : Logic  Operator=NOT  AllPortsSameDT=off  OutDataTypeStr=boolean
  Logical Operator14 : Logic  Operator=OR  Inputs=4  AllPortsSameDT=off  OutDataTypeStr=boolean
  Logical Operator16 : Logic  AllPortsSameDT=off  OutDataTypeStr=boolean
  Logical Operator4 : Logic  AllPortsSameDT=off  OutDataTypeStr=boolean
  Relational Operator1 : RelationalOperator  Operator=>  OutDataTypeStr=boolean  RndMeth=Simplest
  Switch1 : Switch  Criteria=u2 ~= 0
  Switch3 : Switch  Criteria=u2 ~= 0
  Switch6 : Switch  Criteria=u2 ~= 0
  Terminator : Terminator
  Test Detection Criteria1 : hcu_lib/Basic_Blocks/Test Detection Criteria
  Timer2 : hcu_lib/Basic_Blocks/Timer
  Unit Delay1 : UnitDelay  SampleTime=-1  HasFrameUpgradeWarning=on
  VDDM_FrMCU4PreDTC_raw32 : Outport
  VDDM_FrMCU4PreCFS_flg : Outport  Port=2
  wires:
  Logical Operator1/1 -> Logical Operator4/1
  VDDM_FrMCUReady4Pre_flg/1 -> [VDDM_FrMCUReady4Pre_flg]
  [VDDM_FrMCU4PreCFS_flg] -> VDDM_FrMCU4PreCFS_flg/1
  Constant9/1 -> Test Detection Criteria1/3
  [VDDM_FrMCU4PreCFSRls_flg] -> DTC_Couter1/2
  Test Detection Criteria1/1 -> [VDDM_FrMCU4PreDet_flg]  "VDDM_FrMCU4PreDet_flg"
  Logical Operator14/1 -> [VDDM_FrMCU4PreCFSRls_flg]  "VDDM_FrMCU4PreCFSRls_flg"
  Switch1/1 -> Logical Operator13/1, Timer2/2
  [DTC_clear_request] -> Logical Operator14/2
  [VPMM_PowerSta_enum] -> Unit Delay1/1
  Constant14/1 -> Relational Operator1/2
  Equal4/1 -> Switch3/2
  Switch3/1 -> Switch6/3
  [VPMM_PowerSta_enum] -> Equal9/1
  [VDDM_FrMCU4PrePass_flg] -> Logical Operator14/3
  Constant7/1 -> Equal9/2
  Constant29/1 -> Switch6/1
  Unit Delay1/1 -> Equal8/1
  Constant12/1 -> Equal4/2
  Constant17/1 -> Logical Operator14/4
  [task_time_s] -> Test Detection Criteria1/2
  [VDDM_FrMCU4PreCFSRls_flg] -> Switch6/2
  [VDDM_FrMCU4PreDet_flg] -> DTC_Couter1/1
  Constant22/1 -> Equal8/2
  Constant13/1 -> Switch3/3
  Constant3/1 -> DTC_Couter1/3
  Switch6/1 -> Test Detection Criteria1/1
  Equal9/1 -> Logical Operator16/2
  Logical Operator13/1 -> Timer2/1
  DTC_Couter1/2 -> Relational Operator1/1  "VDDM_FrMCU4PreDTC_cnt"
  Constant6/1 -> Switch1/3
  Constant41/1 -> Test Detection Criteria1/4
  [task_time_s] -> Timer2/3
  Equal8/1 -> Logical Operator16/1
  Timer2/1 -> Equal7/1
  Logical Operator16/1 -> Logical Operator14/1
  Equal7/1 -> [VDDM_FrMCU4PrePass_flg]  "VDDM_FrMCU4PrePass_flg"
  [VPMM_PwrStaSW_enum] -> Equal4/1
  [VDDM_FrMCU4PreChk_flg] -> Switch3/1
  Relational Operator1/1 -> Terminator/1  "VDDM_FrMCU4PreDFS_flg"
  Constant28/1 -> Equal7/2
  DTC_Couter1/1 -> [VDDM_FrMCU4PreCFS_flg]  "VDDM_FrMCU4PreCFS_flg"
  Constant18/1 -> Timer2/4
  task_time_s/1 -> [task_time_s]
  VPMM_PwrStaSW_enum/1 -> [VPMM_PwrStaSW_enum]
  VPMM_PowerSta_enum/1 -> [VPMM_PowerSta_enum]
  DTC_clear_request/1 -> [DTC_clear_request]
  Constant/1 -> Equal1/2
  VPMM_PowerUpFault_enum/1 -> Equal1/1
  Equal1/1 -> Logical Operator4/2
  Logical Operator4/1 -> [VDDM_FrMCU4PreChk_flg]
  [VDDM_FrMCU4PrePass_flg] -> DTC_Info/2
  DTC_Info/1 -> VDDM_FrMCU4PreDTC_raw32/1  "VDDM_FrMCU4PreDTC_raw32"
  [VDDM_FrMCU4PreCFS_flg] -> DTC_Info/3
  [VDDM_FrMCU4PreDet_flg] -> DTC_Info/1
  [DTC_clear_request] -> DTC_Info/4
  [VDDM_FrMCUReady4Pre_flg] -> Logical Operator1/1
  [VDDM_FrMCU4PreChk_flg] -> Switch1/1
  Equal2/1 -> Switch1/2
  [VPMM_PwrStaSW_enum] -> Equal2/1
  Constant1/1 -> Equal2/2

== system ddm/DDM/DDM/PMM/power up and power down/HVB ready for precharge fail ==
  note: Diagnostics and Fault Handling
  note: Release Condition After Decision
  note: Test Detection Criteria
  note: Test Pass Criteria
  task_time_s : Inport
  VPMM_PowerSta_enum : Inport  Port=2
  VPMM_PwrStaSW_enum : Inport  Port=3
  VINP_HVBattReady4Pre_enum : Inport  Port=4
  VPMM_PowerUpFault_enum : Inport  Port=5
  DTC_clear_request : Inport  Port=6
  Constant : Constant  Value=ENUM_PUFAULT_PRECHRGCHKFAIL
  Constant12 : Constant  Value=ENUM_PWRSTASW_OFF
  Constant13 : Constant  Value=FALSE
  Constant17 : Constant  Value=KDDM_PwrUpDnDiagnosisOffSW_flg
  Constant18 : Constant  Value=KDDM_HVB4PreDTC_cnt
  Constant2 : Constant  Value=ENUM_PWRSTASW_OFF
  Constant22 : Constant  Value=ENUM_POWERSTA_OFF
  Constant23 : Constant  Value=TRUE
  Constant28 : Constant  Value=KDDM_HVB4PrePassTO_s
  Constant3 : Constant  Value=ENUM_HVBATTREADYPRE_READY
  Constant4 : Constant  Value=ENUM_POWERSTA_STANDBY
  Constant40 : Constant  Value=KDDM_HVB4PreDTC_cnt
  Constant41 : Constant  Value=KDDM_HVB4PreDetTO_s
  Constant5 : Constant  Value=ZERO_INT
  Constant7 : Constant  Value=KDDM_HVB4PrePassTO_s
  Constant9 : Constant  Value=FALSE
  DTC_Couter1 : hcu_lib/Basic_Blocks/DTC_Couter
  DTC_Info : hcu_lib/Basic_Blocks/DTC_Info
  Equal1 : RelationalOperator  Operator=~=  OutDataTypeStr=boolean  RndMeth=Simplest
  Equal2 : RelationalOperator  Operator=~=  OutDataTypeStr=boolean  RndMeth=Simplest
  Equal24 : RelationalOperator  Operator=~=  OutDataTypeStr=boolean  RndMeth=Simplest
  Equal6 : RelationalOperator  OutDataTypeStr=boolean  RndMeth=Simplest
  Equal7 : RelationalOperator  Operator===  OutDataTypeStr=boolean  RndMeth=Simplest
  Equal8 : RelationalOperator  Operator===  OutDataTypeStr=boolean  RndMeth=Simplest
  Equal9 : RelationalOperator  Operator===  OutDataTypeStr=boolean  RndMeth=Simplest
  Logical Operator13 : Logic  Operator=NOT  AllPortsSameDT=off  OutDataTypeStr=boolean
  Logical Operator14 : Logic  Operator=OR  Inputs=4  AllPortsSameDT=off  OutDataTypeStr=boolean
  Logical Operator16 : Logic  AllPortsSameDT=off  OutDataTypeStr=boolean
  Logical Operator4 : Logic  AllPortsSameDT=off  OutDataTypeStr=boolean
  Relational Operator1 : RelationalOperator  Operator=>  OutDataTypeStr=boolean  RndMeth=Simplest
  Switch2 : Switch  Criteria=u2 ~= 0
  Switch3 : Switch  Criteria=u2 ~= 0
  Switch6 : Switch  Criteria=u2 ~= 0
  Terminator : Terminator
  Test Detection Criteria : hcu_lib/Basic_Blocks/Test Detection Criteria
  Timer2 : hcu_lib/Basic_Blocks/Timer
  Unit Delay1 : UnitDelay  SampleTime=-1  HasFrameUpgradeWarning=on
  VDDM_HVB4PreDTC_raw32 : Outport
  VDDM_HVB4PreCFS_flg : Outport  Port=2
  wires:
  [VDDM_HVB4PreCFS_flg] -> VDDM_HVB4PreCFS_flg/1
  Constant23/1 -> Switch2/3
  [VPMM_PwrStaSW_enum] -> Equal2/1
  Constant12/1 -> Equal2/2
  [task_time_s] -> Test Detection Criteria/2
  Switch3/1 -> Switch6/3
  Logical Operator13/1 -> Timer2/1
  Constant28/1 -> Timer2/4
  DTC_Couter1/1 -> [VDDM_HVB4PreCFS_flg]  "VDDM_HVB4PreCFS_flg"
  Equal6/1 -> [VDDM_HVB4PrePass_flg]  "VDDM_HVB4PrePass_flg"
  [DTC_clear_request] -> Logical Operator14/2
  [VPMM_PowerSta_enum] -> Unit Delay1/1
  Constant40/1 -> Test Detection Criteria/3
  [VDDM_HVB4PreChk_flg] -> Switch3/1
  Equal2/1 -> Switch3/2
  Switch2/1 -> Logical Operator13/1, Timer2/2
  [VPMM_PowerSta_enum] -> Equal9/1
  Test Detection Criteria/1 -> [VDDM_HVB4PreDet_flg]  "VDDM_HVB4PreDet_flg"
  Unit Delay1/1 -> Equal7/1
  Logical Operator16/1 -> Logical Operator14/1
  Equal7/1 -> Logical Operator16/1
  Switch6/1 -> Test Detection Criteria/1
  Constant17/1 -> Logical Operator14/4
  [task_time_s] -> Timer2/3
  Logical Operator14/1 -> [VDDM_HVB4PreCFSRls_flg]  "VDDM_HVB4PreCFSRls_flg"
  Constant13/1 -> Switch3/3
  [VDDM_HVB4PrePass_flg] -> Logical Operator14/3
  Constant4/1 -> Equal9/2
  Constant5/1 -> Relational Operator1/2
  Equal9/1 -> Logical Operator16/2
  Constant18/1 -> DTC_Couter1/3
  Constant22/1 -> Equal7/2
  [VDDM_HVB4PreCFSRls_flg] -> DTC_Couter1/2
  Relational Operator1/1 -> Terminator/1  "VDDM_HVB4PreDFS_flg"
  DTC_Couter1/2 -> Relational Operator1/1  "VDDM_HVB4PreDTC_cnt"
  Constant9/1 -> Switch6/1
  [VDDM_HVB4PreCFSRls_flg] -> Switch6/2
  Constant41/1 -> Test Detection Criteria/4
  [VDDM_HVB4PreDet_flg] -> DTC_Couter1/1
  Timer2/1 -> Equal6/1
  Constant7/1 -> Equal6/2
  VPMM_PowerSta_enum/1 -> [VPMM_PowerSta_enum]
  VPMM_PwrStaSW_enum/1 -> [VPMM_PwrStaSW_enum]
  task_time_s/1 -> [task_time_s]
  Constant3/1 -> Equal24/2
  VINP_HVBattReady4Pre_enum/1 -> Equal24/1
  DTC_clear_request/1 -> [DTC_clear_request]
  Constant/1 -> Equal8/2
  VPMM_PowerUpFault_enum/1 -> Equal8/1
  Equal24/1 -> Logical Operator4/1
  Equal8/1 -> Logical Operator4/2
  Logical Operator4/1 -> [VDDM_HVB4PreChk_flg]
  DTC_Info/1 -> VDDM_HVB4PreDTC_raw32/1  "VDDM_HVB4PreDTC_raw32"
  [VDDM_HVB4PreCFS_flg] -> DTC_Info/3
  [VDDM_HVB4PrePass_flg] -> DTC_Info/2
  [VDDM_HVB4PreDet_flg] -> DTC_Info/1
  [DTC_clear_request] -> DTC_Info/4
  [VPMM_PwrStaSW_enum] -> Equal1/1
  [VDDM_HVB4PreChk_flg] -> Switch2/1
  Constant2/1 -> Equal1/2
  Equal1/1 -> Switch2/2

== system ddm/DDM/DDM/PMM/power up and power down/High level system safety check fail ==
  note: Diagnostics and Fault Handling
  note: Test Detection Criteria
  note: Release Condition After Decision
  note: Test Pass Criteria
  task_time_s : Inport
  VPMM_PowerSta_enum : Inport  Port=2
  VPMM_PwrStaSW_enum : Inport  Port=3
  VPMM_SafetyChkHLv_flg : Inport  Port=4
  VPMM_PowerUpFault_enum : Inport  Port=5
  DTC_clear_request : Inport  Port=6
  Constant : Constant  Value=ENUM_PUFAULT_SAFETYCHKFAIL
  Constant1 : Constant  Value=ENUM_PWRSTASW_OFF
  Constant12 : Constant  Value=ENUM_PWRSTASW_OFF
  Constant13 : Constant  Value=FALSE
  Constant14 : Constant  Value=ZERO_INT
  Constant17 : Constant  Value=KDDM_PwrUpDnDiagnosisOffSW_flg
  Constant18 : Constant  Value=KDDM_HiLvSaChkPassTO_s
  Constant22 : Constant  Value=ENUM_POWERSTA_OFF
  Constant28 : Constant  Value=KDDM_HiLvSaChkPassTO_s
  Constant29 : Constant  Value=FALSE
  Constant3 : Constant  Value=KDDM_HiLvSaChkDTC_cnt
  Constant41 : Constant  Value=KDDM_HiLvSaChkDetTO_s
  Constant6 : Constant  Value=TRUE
  Constant7 : Constant  Value=ENUM_POWERSTA_STANDBY
  Constant9 : Constant  Value=KDDM_HiLvSaChkDTC_cnt
  DTC_Couter1 : hcu_lib/Basic_Blocks/DTC_Couter
  DTC_Info : hcu_lib/Basic_Blocks/DTC_Info
  Equal1 : RelationalOperator  Operator===  OutDataTypeStr=boolean  RndMeth=Simplest
  Equal2 : RelationalOperator  Operator=~=  OutDataTypeStr=boolean  RndMeth=Simplest
  Equal4 : RelationalOperator  Operator=~=  OutDataTypeStr=boolean  RndMeth=Simplest
  Equal7 : RelationalOperator  OutDataTypeStr=boolean  RndMeth=Simplest
  Equal8 : RelationalOperator  Operator===  OutDataTypeStr=boolean  RndMeth=Simplest
  Equal9 : RelationalOperator  Operator===  OutDataTypeStr=boolean  RndMeth=Simplest
  Logical Operator13 : Logic  Operator=NOT  AllPortsSameDT=off  OutDataTypeStr=boolean
  Logical Operator14 : Logic  Operator=OR  Inputs=4  AllPortsSameDT=off  OutDataTypeStr=boolean
  Logical Operator16 : Logic  AllPortsSameDT=off  OutDataTypeStr=boolean
  Logical Operator4 : Logic  Operator=NOT  AllPortsSameDT=off  OutDataTypeStr=boolean
  Logical Operator5 : Logic  AllPortsSameDT=off  OutDataTypeStr=boolean
  Relational Operator1 : RelationalOperator  Operator=>  OutDataTypeStr=boolean  RndMeth=Simplest
  Switch1 : Switch  Criteria=u2 ~= 0
  Switch3 : Switch  Criteria=u2 ~= 0
  Switch6 : Switch  Criteria=u2 ~= 0
  Terminator : Terminator
  Test Detection Criteria1 : hcu_lib/Basic_Blocks/Test Detection Criteria
  Timer2 : hcu_lib/Basic_Blocks/Timer
  Unit Delay1 : UnitDelay  SampleTime=-1  HasFrameUpgradeWarning=on
  VDDM_HiLvSaChkDTC_raw32 : Outport
  VDDM_HiLvSaChkCFS_flg : Outport  Port=2
  wires:
  [VDDM_HiLvSaChkCFS_flg] -> VDDM_HiLvSaChkCFS_flg/1
  Equal4/1 -> Switch3/2
  Constant9/1 -> Test Detection Criteria1/3
  Logical Operator14/1 -> [VDDM_HiLvSaChkCFSRls_flg]  "VDDM_HiLvSaChkCFSRls_flg"
  Logical Operator16/1 -> Logical Operator14/1
  Constant28/1 -> Equal7/2
  Constant3/1 -> DTC_Couter1/3
  Constant18/1 -> Timer2/4
  [VDDM_HiLvSaChkChk_flg] -> Switch3/1
  DTC_Couter1/1 -> [VDDM_HiLvSaChkCFS_flg]  "VDDM_HiLvSaChkCFS_flg"
  Test Detection Criteria1/1 -> [VDDM_HiLvSaChkDet_flg]  "VDDM_HiLvSaChkDet_flg"
  Constant41/1 -> Test Detection Criteria1/4
  [VDDM_HiLvSaChkCFSRls_flg] -> DTC_Couter1/2
  [VDDM_HiLvSaChkCFSRls_flg] -> Switch6/2
  [VDDM_HiLvSaChkDet_flg] -> DTC_Couter1/1
  Equal2/1 -> Switch1/2
  Constant12/1 -> Equal4/2
  Equal8/1 -> Logical Operator16/1
  Logical Operator13/1 -> Timer2/1
  Constant17/1 -> Logical Operator14/4
  [task_time_s] -> Timer2/3
  DTC_Couter1/2 -> Relational Operator1/1  "VDDM_HiLvSaChkDTC_cnt"
  Switch6/1 -> Test Detection Criteria1/1
  [VPMM_PowerSta_enum] -> Unit Delay1/1
  Timer2/1 -> Equal7/1
  [VPMM_PowerSta_enum] -> Equal9/1
  Constant22/1 -> Equal8/2
  Unit Delay1/1 -> Equal8/1
  Equal9/1 -> Logical Operator16/2
  Constant7/1 -> Equal9/2
  Equal7/1 -> [VDDM_HiLvSaChkPass_flg]  "VDDM_HiLvSaChkPass_flg"
  Constant14/1 -> Relational Operator1/2
  [task_time_s] -> Test Detection Criteria1/2
  Constant29/1 -> Switch6/1
  Switch3/1 -> Switch6/3
  Switch1/1 -> Logical Operator13/1, Timer2/2
  [DTC_clear_request] -> Logical Operator14/2
  Constant13/1 -> Switch3/3
  [VDDM_HiLvSaChkPass_flg] -> Logical Operator14/3
  Constant6/1 -> Switch1/3
  [VPMM_PwrStaSW_enum] -> Equal4/1
  Relational Operator1/1 -> Terminator/1  "VDDM_HiLvSaChkDFS_flg"
  Logical Operator5/1 -> [VDDM_HiLvSaChkChk_flg]
  VPMM_PowerUpFault_enum/1 -> Equal1/1
  VPMM_SafetyChkHLv_flg/1 -> Logical Operator4/1
  Logical Operator4/1 -> Logical Operator5/1
  Equal1/1 -> Logical Operator5/2
  Constant/1 -> Equal1/2
  DTC_clear_request/1 -> [DTC_clear_request]
  VPMM_PowerSta_enum/1 -> [VPMM_PowerSta_enum]
  VPMM_PwrStaSW_enum/1 -> [VPMM_PwrStaSW_enum]
  task_time_s/1 -> [task_time_s]
  DTC_Info/1 -> VDDM_HiLvSaChkDTC_raw32/1  "VDDM_HiLvSaChkDTC_raw32"
  [VDDM_HiLvSaChkPass_flg] -> DTC_Info/2
  [VDDM_HiLvSaChkCFS_flg] -> DTC_Info/3
  [VDDM_HiLvSaChkDet_flg] -> DTC_Info/1
  [DTC_clear_request] -> DTC_Info/4
  Constant1/1 -> Equal2/2
  [VPMM_PwrStaSW_enum] -> Equal2/1
  [VDDM_HiLvSaChkChk_flg] -> Switch1/1
